simulink model "SS_F16_Block_ACC"  (Simulink 8.9)
settings: Solver=ode5  StartTime=0.0  StopTime=30.0  FixedStep=deltaT  RelTol=1e-3  EnableMultiTasking=on
values from neighbouring files (symbols this model uses):
  A = A_lo    [runLINF16sim.m]    (also in runLINF16sim_ACC.m; variables_chpt5.mat = [0 0 0 0 0 0 0 0 0 0 0 0 ... (324 elements, 18x18)])
  B = B_lo    [runLINF16sim.m]    (also in runLINF16sim_ACC.m; variables_chpt5.mat = [0 0 0 0 0 0 0 0 0 0 0 0 ... (72 elements, 18x4)])
  C = C_lo    [runLINF16sim.m]    (also in runLINF16sim_ACC.m; variables_chpt5.mat = [1 0 0 0 0 0 0 0 0 0 0 0 ... (342 elements, 19x18)])
  D = D_lo    [runLINF16sim.m]    (also in runLINF16sim_ACC.m; variables_chpt5.mat = [0 0 0 0 0 0 0 0 0 0 0 0 ... (76 elements, 19x4)])
  DisAil_1 = AileronDis    (= 0)    [runF16Sim.m]    (also in runLINF16sim.m; runLINF16sim_ACC.m; variables_chpt5.mat)
  DisAil_2 = -2*AileronDis    (= 0)    [runF16Sim.m]    (also in runLINF16sim.m; runLINF16sim_ACC.m; variables_chpt5.mat)
  DisAil_3 = AileronDis    (= 0)    [runF16Sim.m]    (also in runLINF16sim.m; runLINF16sim_ACC.m; variables_chpt5.mat)
  DisEle_1 = ElevatorDis    (= 0)    [runF16Sim.m]    (also in runLINF16sim.m; runLINF16sim_ACC.m; variables_chpt5.mat)
  DisEle_2 = -2*ElevatorDis    (= 0)    [runF16Sim.m]    (also in runLINF16sim.m; runLINF16sim_ACC.m; variables_chpt5.mat)
  DisEle_3 = ElevatorDis    (= 0)    [runF16Sim.m]    (also in runLINF16sim.m; runLINF16sim_ACC.m; variables_chpt5.mat)
  DisRud_1 = RudderDis    (= 0)    [runF16Sim.m]    (also in runLINF16sim.m; runLINF16sim_ACC.m; variables_chpt5.mat)
  DisRud_2 = -2*RudderDis    (= 0)    [runF16Sim.m]    (also in runLINF16sim.m; runLINF16sim_ACC.m; variables_chpt5.mat)
  DisRud_3 = RudderDis    (= 0)    [runF16Sim.m]    (also in runLINF16sim.m; runLINF16sim_ACC.m; variables_chpt5.mat)
  gD = 9.80665    [FindF16Dynamics_ACC.m]    (also in runLINF16sim_ACC.m; variables_chpt5.mat)
  thrust = 5000    [FindF16Dynamics.m]    (also in FindF16Dynamics_ACC.m; runF16Sim.m; runLINF16sim.m = 0; runLINF16sim_ACC.m = 0)
  trim_control = trim_control_lo    [runLINF16sim.m]    (also in runLINF16sim_ACC.m; trim_F16_ACC.m = [UX(2);UX(4);UX(5)]; variables_chpt5.mat = [-2.46068617229 2.91286693087e-16 2.79661206579e-15])
  trim_state = xu_lo    [runLINF16sim.m]    (also in runLINF16sim_ACC.m; trim_F16_ACC.m = xu(1:12); variables_chpt5.mat = [0 0 15000 0 0.0779375118365 0 500 0.0779375118365 0 0 0 0 .)
  trim_thrust = trim_thrust_lo    [runLINF16sim.m]    (also in runLINF16sim_ACC.m; trim_F16_ACC.m = UX(1); variables_chpt5.mat = 2120.62144782)
  xa = 0    [FindF16Dynamics_ACC.m]    (also in runLINF16sim_ACC.m = 5; variables_chpt5.mat = 5)
settings Model: Creator=russ1110  LastModifiedBy=Lukas  ExtModeAutoUpdateStatusClock=off
settings DataIOCC: SignalLoggingName=sigsOut
settings OptimizationCC: BooleanDataType=off  LifeSpan=auto
settings DebuggingCC: SaveWithParameterizedLinksMsg=none  SignalResolutionControl=TryResolveAllWithWarning  MultiTaskDSMMsg=warning  MultiTaskCondExecSysMsg=none  FcnCallInpInsideContextMsg=error  StateNameClashWarn=none  SFUnexpectedBacktrackingDiag=error  SFNoUnconditionalDefaultTransitionDiag=error  SFExecutionAtInitializationDiag=warning
settings HardwareCC: TargetUnknown=on
settings GRTTargetCC: GeneratePreprocessorConditionals=Use local settings

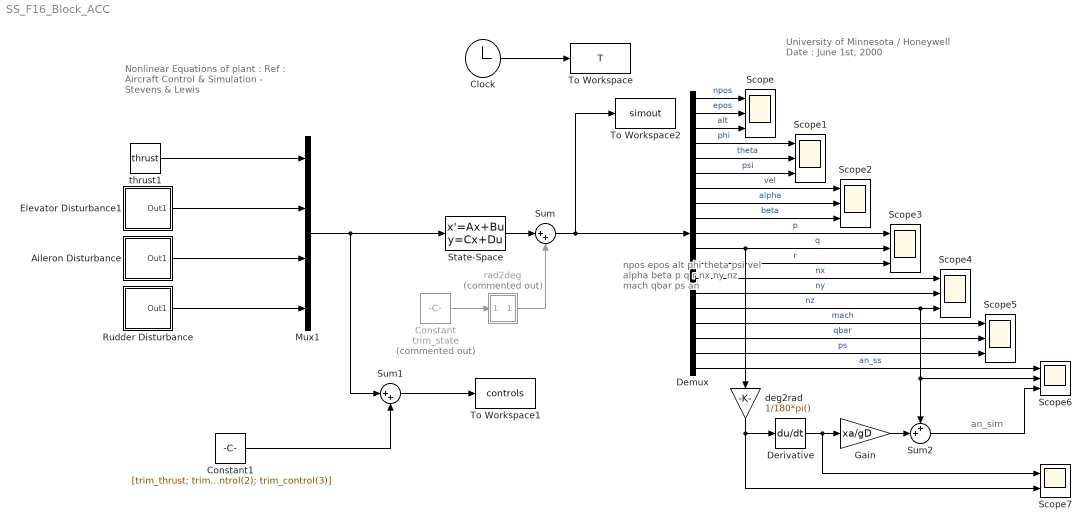
== system SS_F16_Block_ACC ==
  note: an_sim
  note: npos
      | epos
      | alt
      | phi
      | theta
      | psi
      | vel
      | alpha
      | beta
      | p
      | q
      | r
      | nx
      | ny
      | nz
      | mach
      | qbar
      | ps
      | an
  note: University of Minnesota / Honeywell
      | Date : June 1st, 2000
  note: Nonlinear Equations of plant :
      | Ref : Aircraft Control & Simulation
      | - Stevens & Lewis
  Aileron Disturbance : Subsystem
  Clock : Clock
      settings: Decimation=50
  Constant : Constant  Commented=on  Value=trim_state
  Constant1 : Constant  Value=[trim_thrust; trim_control(1); trim_control(2); trim_control(3)]
  Demux : Demux  Outputs=19
  Derivative : Derivative
  Elevator Disturbance1 : Subsystem
  Gain : Gain  Gain=xa/gD
  Mux1 : Mux
  Rudder Disturbance : Subsystem
  Scope{,1..6} (7 alike) : Scope  NumInputPorts=3
  Scope7 : Scope  NumInputPorts=2
  State-Space : StateSpace  A=A  B=B  C=C  D=D  X0=0
  Sum : Sum  Inputs=|++  SaturateOnIntegerOverflow=on  InputSameDT=on  OutDataTypeStr=Inherit: Same as first input
  Sum1 : Sum  Inputs=|++  SaturateOnIntegerOverflow=on  InputSameDT=on  OutDataTypeStr=Inherit: Same as first input
  Sum2 : Sum  Inputs=++|
  To Workspace : ToWorkspace  VariableName=T  SampleTime=-1
      settings: Decimation=100
  To Workspace1 : ToWorkspace  VariableName=controls  SampleTime=-1
      settings: Decimation=100
  To Workspace2 : ToWorkspace  VariableName=simout  SampleTime=-1
      settings: Decimation=100
  deg2rad : Gain  Gain=1/180*pi()
  rad2deg : Subsystem  Commented=on
  thrust1 : Constant  Value=thrust  VectorParams1D=off
  wires:
  Clock/1 -> To Workspace/1
  Demux/1 -> Scope/1  "npos"
  Demux/2 -> Scope/2  "epos"
  Demux/3 -> Scope/3  "alt"
  Demux/5 -> Scope1/2  "theta"
  Demux/6 -> Scope1/3  "psi"
  Demux/7 -> Scope2/1  "vel"
  Demux/8 -> Scope2/2  "alpha"
  Demux/9 -> Scope2/3  "beta"
  Demux/10 -> Scope3/1  "p"
  Demux/11 -> Scope3/2, deg2rad/1  "q"
  Demux/12 -> Scope3/3  "r"
  Demux/13 -> Scope4/1  "nx"
  Demux/14 -> Scope4/2  "ny"
  Demux/4 -> Scope1/1  "phi"
  Demux/16 -> Scope5/1  "mach"
  Demux/17 -> Scope5/2  "qbar"
  Demux/18 -> Scope5/3  "ps"
  State-Space/1 -> Sum/1
  Sum/1 -> Demux/1, To Workspace2/1
  thrust1/1 -> Mux1/1
  Elevator Disturbance1/1(Out1) -> Mux1/2
  Aileron Disturbance/1(Out1) -> Mux1/3
  Rudder Disturbance/1(Out1) -> Mux1/4
  Constant1/1 -> Sum1/2
  Mux1/1 -> State-Space/1, Sum1/1
  Sum1/1 -> To Workspace1/1
  rad2deg/1(Out1) -> Sum/2
  Constant/1 -> rad2deg/1(In1)
  Demux/19 -> Scope6/1  "an_ss"
  Demux/15 -> Scope4/3, Scope6/2, Sum2/1  "nz"
  Sum2/1 -> Scope6/3
  Gain/1 -> Sum2/2
  Derivative/1 -> Scope7/1, Gain/1
  deg2rad/1 -> Derivative/1, Scope7/2

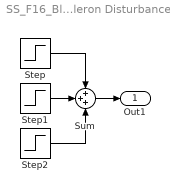
== system SS_F16_Block_ACC/Aileron Disturbance ==
  Step : Step  After=DisAil_1  SampleTime=0
  Step1 : Step  Time=3  After=DisAil_2  SampleTime=0
  Step2 : Step  Time=5  After=DisAil_3  SampleTime=0
  Sum : Sum  Inputs=+++  SaturateOnIntegerOverflow=on  InputSameDT=on  OutDataTypeStr=Inherit: Same as first input
  Out1 : Outport
  wires:
  Step1/1 -> Sum/2
  Step/1 -> Sum/1
  Step2/1 -> Sum/3
  Sum/1 -> Out1/1

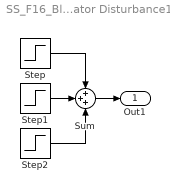
== system SS_F16_Block_ACC/Elevator Disturbance1 ==
  Step : Step  After=DisEle_1  SampleTime=0
  Step1 : Step  Time=3  After=DisEle_2  SampleTime=0
  Step2 : Step  Time=5  After=DisEle_3  SampleTime=0
  Sum : Sum  Inputs=+++  SaturateOnIntegerOverflow=on  InputSameDT=on  OutDataTypeStr=Inherit: Same as first input
  Out1 : Outport
  wires:
  Step1/1 -> Sum/2
  Step/1 -> Sum/1
  Step2/1 -> Sum/3
  Sum/1 -> Out1/1

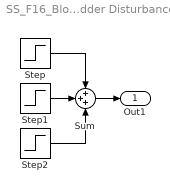
== system SS_F16_Block_ACC/Rudder Disturbance ==
  Step : Step  After=DisRud_1  SampleTime=0
  Step1 : Step  Time=1.5  After=DisRud_2  SampleTime=0
  Step2 : Step  Time=2  After=DisRud_3  SampleTime=0
  Sum : Sum  Inputs=+++  SaturateOnIntegerOverflow=on  InputSameDT=on  OutDataTypeStr=Inherit: Same as first input
  Out1 : Outport
  wires:
  Step1/1 -> Sum/2
  Step/1 -> Sum/1
  Step2/1 -> Sum/3
  Sum/1 -> Out1/1

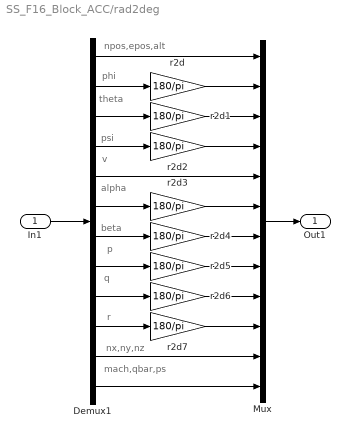
== system SS_F16_Block_ACC/rad2deg ==
  note: npos,epos,alt
  note: phi
  note: theta
  note: psi
  note: v
  note: alpha
  note: beta
  note: p
  note: q
  note: r
  note: nx,ny,nz
  note: mach,qbar,ps
  In1 : Inport
  Demux1 : Demux  Outputs=[3 1 1 1 1 1 1 1 1 1 3 3]
  Mux : Mux  Inputs=[3 1 1 1 1 1 1 1 1 1 3 3]
  r2d{,1..7} (8 alike) : Gain  Gain=180/pi  SaturateOnIntegerOverflow=on  OutDataTypeStr=Inherit: Same as input  ParamDataTypeStr=Inherit: Same as input
  Out1 : Outport
  wires:
  In1/1 -> Demux1/1
  Demux1/2 -> r2d/1
  Demux1/3 -> r2d1/1
  Demux1/4 -> r2d2/1
  Demux1/1 -> Mux/1
  Demux1/5 -> Mux/5
  r2d2/1 -> Mux/4
  r2d1/1 -> Mux/3
  r2d/1 -> Mux/2
  Demux1/6 -> r2d3/1
  Demux1/7 -> r2d4/1
  Demux1/8 -> r2d5/1
  Demux1/9 -> r2d6/1
  Demux1/10 -> r2d7/1
  r2d3/1 -> Mux/6
  r2d4/1 -> Mux/7
  r2d5/1 -> Mux/8
  r2d6/1 -> Mux/9
  r2d7/1 -> Mux/10
  Mux/1 -> Out1/1
  Demux1/11 -> Mux/11
  Demux1/12 -> Mux/12
